simulink model "MagnetSystemTuning"  (R2020b)
settings: Solver=VariableStepAuto  StartTime=0.0  StopTime=1  FixedStep=0.001  RelTol=1e-3
values from neighbouring files (symbols this model uses):
  A = [0, dfdx/m, dfdi/m ... (first row only)    [magnetABCD.m]
  B = [0 ... (first row only)    [magnetABCD.m]
  C = zeros(2,3)    [magnetABCD.m]
undefined symbols (not defined in the file or in its folder): coeffLQR, coeffPP, current, F, initialConditions, initialConditionsOBS, intensityVariance, KoLQR, LL, positions, positionsVariance, target
libraries: simulink x1
settings Model: Creator=paolo  LastModifiedBy=paolo
settings SolverCC: ZeroCrossAlgorithm=Adaptive
settings DebuggingCC: IgnoredZcDiagnostic=none

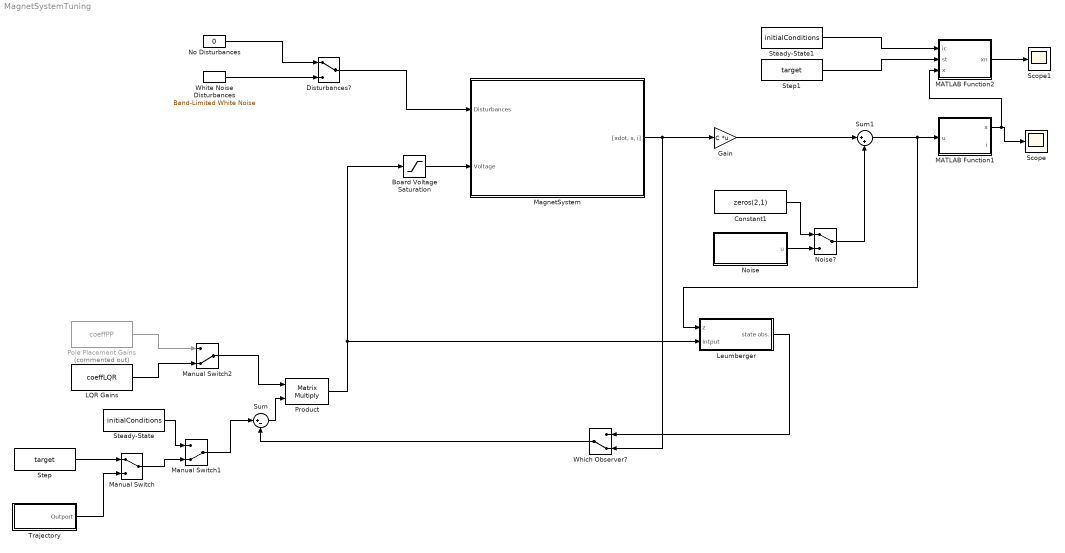
== system MagnetSystemTuning ==
  Board Voltage Saturation : Saturate  UpperLimit=15  LowerLimit=0.1
  Constant1 : Constant  Value=zeros(2,1)
  Disturbances? : ManualSwitch
  Gain : Gain  Gain=C  Multiplication=Matrix(K*u)
  LQR Gains : Constant  Value=coeffLQR  VectorParams1D=off
  Leumberger : Subsystem
  MATLAB Function1 : MATLAB Function  TreatAsAtomicUnit=on
  MATLAB Function2 : MATLAB Function  TreatAsAtomicUnit=on
  MagnetSystem : Subsystem
  Manual Switch : ManualSwitch
  Manual Switch1 : ManualSwitch  CurrentSetting=0
  Manual Switch2 : ManualSwitch  CurrentSetting=0
  No Disturbances : Constant  Value=0
  Noise : Subsystem
  Noise? : ManualSwitch
  Pole Placement Gains : Constant  Commented=on  Value=coeffPP  VectorParams1D=off
  Product : Product  Multiplication=Matrix(*)
  Scope : Scope
  Scope1 : Scope
  Steady-State : Constant  Value=initialConditions  VectorParams1D=off
  Steady-State1 : Constant  Value=initialConditions  VectorParams1D=off
  Step : Constant  Value=target  VectorParams1D=off
  Step1 : Constant  Value=target  VectorParams1D=off
  Sum : Sum  Inputs=|+-
  Sum1 : Sum  Inputs=|++
  Trajectory : Subsystem
  Which Observer? : ManualSwitch  CurrentSetting=0
  White Noise Disturbances : simulink/Sources/Band-Limited White Noise  Cov=[0.1]  Ts=0.1  seed=[23341]
  wires:
  Board Voltage Saturation/1 -> MagnetSystem/2(Voltage)
  MagnetSystem/1("[xdot, x, i]") -> Which Observer?/2, Gain/1
  Steady-State/1 -> Manual Switch1/1
  Sum/1 -> Product/2
  No Disturbances/1 -> Disturbances?/1
  Disturbances?/1 -> MagnetSystem/1(Disturbances)
  White Noise Disturbances/1 -> Disturbances?/2
  Manual Switch1/1 -> Sum/1
  Product/1 -> Board Voltage Saturation/1, Leumberger/2(Intput)
  Manual Switch2/1 -> Product/1
  LQR Gains/1 -> Manual Switch2/2
  Pole Placement Gains/1 -> Manual Switch2/1
  Leumberger/1(state obs.) -> Which Observer?/1
  Which Observer?/1 -> Sum/2
  Gain/1 -> Sum1/1
  Noise?/1 -> Sum1/2
  Noise/1(u) -> Noise?/2
  Sum1/1 -> Leumberger/1(z), MATLAB Function1/1(u)
  Constant1/1 -> Noise?/1
  Step/1 -> Manual Switch/1
  Manual Switch/1 -> Manual Switch1/2
  Trajectory/1(Outport) -> Manual Switch/2
  MATLAB Function1/1(x) -> MATLAB Function2/3(x), Scope/1
  Steady-State1/1 -> MATLAB Function2/1(ic)
  Step1/1 -> MATLAB Function2/2(st)
  MATLAB Function2/1(xn) -> Scope1/1

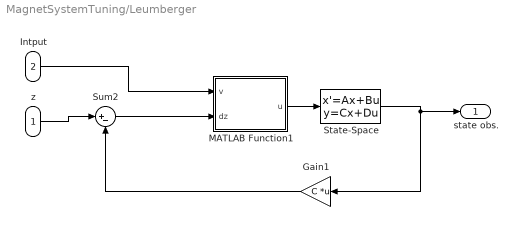
== system MagnetSystemTuning/Leumberger ==
  z : Inport
  Intput : Inport  Port=2
  Gain1 : Gain  Gain=C  Multiplication=Matrix(K*u)
  MATLAB Function1 : MATLAB Function  TreatAsAtomicUnit=on
  State-Space : StateSpace  A=A  B=[B KoLQR]  C=eye(3)  D=zeros(3,3)  InitialCondition=initialConditionsOBS
  Sum2 : Sum  Inputs=|+-
  state obs. : Outport
  wires:
  z/1 -> Sum2/1
  State-Space/1 -> Gain1/1, state obs./1
  Gain1/1 -> Sum2/2
  Sum2/1 -> MATLAB Function1/2(dz)
  Intput/1 -> MATLAB Function1/1(v)
  MATLAB Function1/1(u) -> State-Space/1

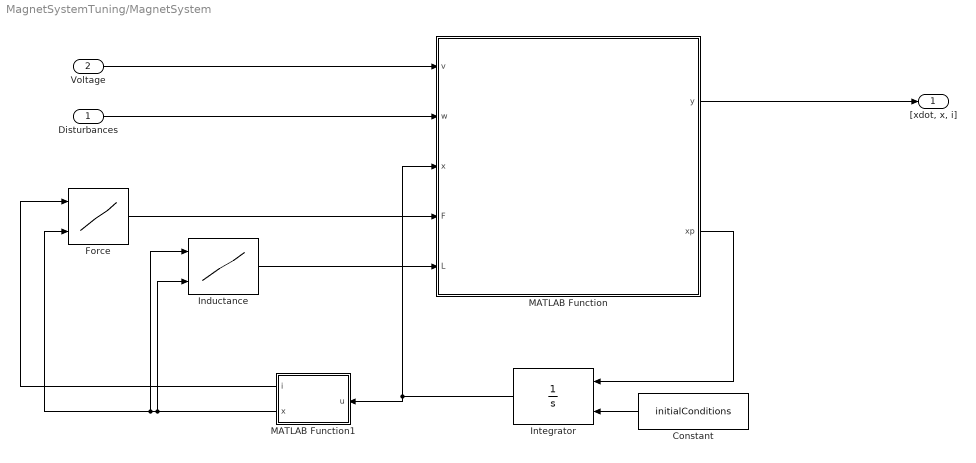
== system MagnetSystemTuning/MagnetSystem ==
  Disturbances : Inport
  Voltage : Inport  Port=2
  Constant : Constant  Value=initialConditions
  Force : Lookup_n-D  BreakpointsForDimension1=current  BreakpointsForDimension2=positions  Table=F  InternalRulePriority=Speed  RndMeth=Simplest  InputSameDT=on
      settings: InputPortMap=u0,u1
  Inductance : Lookup_n-D  BreakpointsForDimension1=current  BreakpointsForDimension2=positions  Table=LL  InternalRulePriority=Speed  RndMeth=Simplest  InputSameDT=on
      settings: InputPortMap=u0,u1
  Integrator : Integrator  InitialConditionSource=external
  MATLAB Function : MATLAB Function  TreatAsAtomicUnit=on
  MATLAB Function1 : MATLAB Function  TreatAsAtomicUnit=on
  "[xdot, x, i]" : Outport
  wires:
  Integrator/1 -> MATLAB Function1/1(u), MATLAB Function/3(x)
  Voltage/1 -> MATLAB Function/1(v)
  Constant/1 -> Integrator/2
  Disturbances/1 -> MATLAB Function/2(w)
  MATLAB Function/1(y) -> "[xdot, x, i]"/1
  MATLAB Function/2(xp) -> Integrator/1
  MATLAB Function1/1(i) -> Force/1
  MATLAB Function1/2(x) -> Inductance/2, Force/2, Inductance/1
  Inductance/1 -> MATLAB Function/5(L)
  Force/1 -> MATLAB Function/4(F)

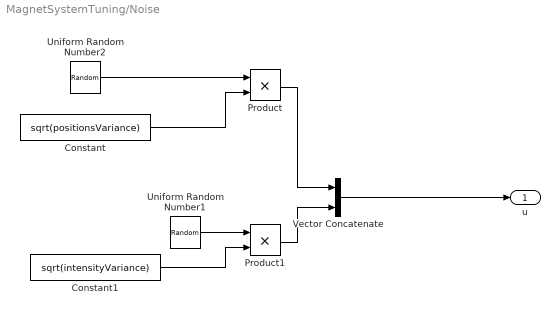
== system MagnetSystemTuning/Noise ==
  Constant : Constant  Value=sqrt(positionsVariance)
  Constant1 : Constant  Value=sqrt(intensityVariance)
  Product : Product
  Product1 : Product
  Uniform Random Number1 : UniformRandomNumber  SampleTime=0.001
  Uniform Random Number2 : UniformRandomNumber  SampleTime=0.001
  Vector Concatenate : Concatenate  Mode=Multidimensional array
  u : Outport
  wires:
  Constant1/1 -> Product1/2
  Vector Concatenate/1 -> u/1
  Constant/1 -> Product/2
  Product1/1 -> Vector Concatenate/2
  Product/1 -> Vector Concatenate/1
  Uniform Random Number2/1 -> Product/1
  Uniform Random Number1/1 -> Product1/1

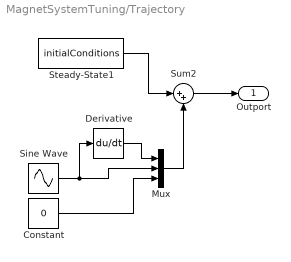
== system MagnetSystemTuning/Trajectory ==
  Constant : Constant  Value=0
  Derivative : Derivative
  Mux : Mux  Inputs=3
  Sine Wave : Sin  Amplitude=0.0002  Frequency=5  SampleTime=0
  Steady-State1 : Constant  Value=initialConditions  VectorParams1D=off
  Sum2 : Sum  Inputs=|++
  Outport : Outport
  wires:
  Steady-State1/1 -> Sum2/1
  Sum2/1 -> Outport/1
  Derivative/1 -> Mux/1
  Mux/1 -> Sum2/2
  Constant/1 -> Mux/3
  Sine Wave/1 -> Derivative/1, Mux/2

== matlab function MagnetSystemTuning/MagnetSystem/MATLAB Function1 ==
  data: i output; u input; x output
function [i, x] = fcn(u)
x = u(2);
i = u(3);

== matlab function MagnetSystemTuning/MagnetSystem/MATLAB Function ==
  data: v input; y output; w input; x input; xp output; F input; L input
function [y,xp] = fcn(v,w,x,F,L)

R = 4.1;
m = 0.8766;
g = 9.81;

x1 = x(1);
x2 = x(2);
x3 = x(3);

xp = [((F/m)-g);x1;((v+w)-R*x3)/L];
y = [x1;x2;x3];

== matlab function MagnetSystemTuning/MATLAB Function1 ==
  data: x output; i output; u input
function [x, i] = fcn(u)
x = u(1);
i = u(2);

== matlab function MagnetSystemTuning/Leumberger/MATLAB Function1 ==
  data: u output; v input; dz input
function u  = fcn(v,dz)
ut = [v, dz(1), dz(2)];
u = ut';

== matlab function MagnetSystemTuning/MATLAB Function2 ==
  data: xn output; ic input; st input; x input
function xn  = fcn(ic, st, x)
xn = (x - ic(2)) / (st(2) - ic(2));
